simulink model "ACFT"  (R2024b)
settings: Solver=ode1  StartTime=0.0  StopTime=10.0  FixedStep=0.01  RelTol=1e-3
undefined symbols (not defined in the file): Inertia
libraries: Aerodynamics x1, Atmospheric x1, EqM x1, Propulsion x1
settings Model: Creator=ada09  LastModifiedBy=ada09
settings DataIOCC: SaveState=on  ReturnWorkspaceOutputs=off

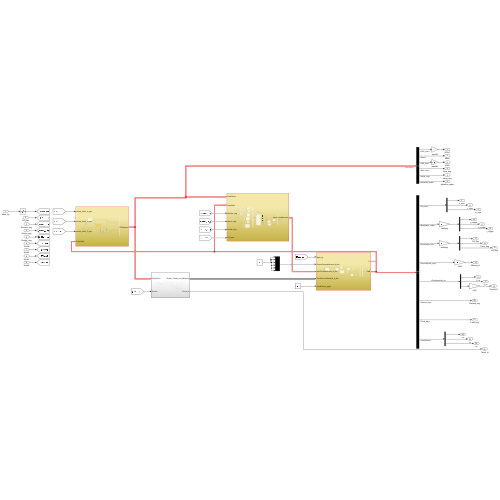
[thumbnail: Simulink's stored preview of the top-level diagram]
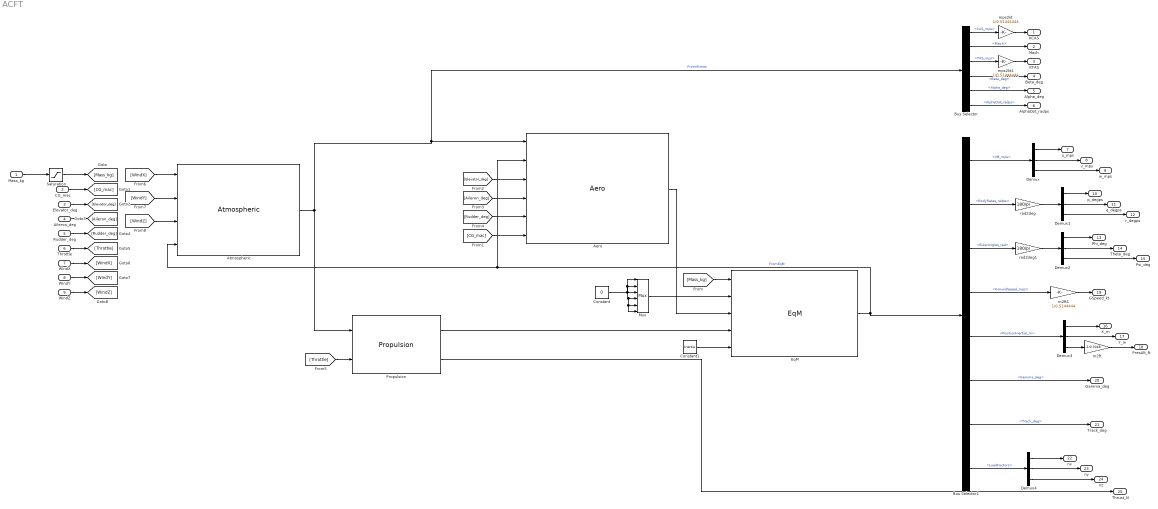
== system ACFT ==
  Mass_kg : Inport
  CG_mac : Inport  Port=2
  Elevator_deg : Inport  Port=3
  Aileron_deg : Inport  Port=4
  Rudder_deg : Inport  Port=5
  Throttle : Inport  Port=6
  WindX : Inport  Port=7
  WindY : Inport  Port=8
  WindZ : Inport  Port=9
  Aero : Aerodynamics/Aero  SystemSampleTime=-1  VariantActivationTime=update diagram  AllowFlexibleInterface=on  Latency=0  AutoFrameSizeCalculation=off
  Atmospheric : Atmospheric/Atmospheric  SystemSampleTime=-1  VariantActivationTime=update diagram  AllowFlexibleInterface=on  Latency=0  AutoFrameSizeCalculation=off
  Bus Selector : BusSelector  OutputSignals=CAS_mps,Mach,TAS_mps,Beta_deg,Alpha_deg,AlphaDot_radps
  Bus Selector1 : BusSelector  OutputSignals=VB_mps,BodyRates_radps,EulerAngles_rad,GroundSpeed_mps,PositionInertial_m,Gamma_deg,Track_deg,LoadFactors
  Constant : Constant  Value=0
  Constant1 : Constant  Value=Inertia
  Demux{,1..4} (5 alike) : Demux  Outputs=3
  EqM : EqM/EqM  SystemSampleTime=-1  VariantActivationTime=update diagram  AllowFlexibleInterface=on  Latency=0  AutoFrameSizeCalculation=off
  Mux : Mux  Inputs=6
  Propulsion : Propulsion/Propulsion  SystemSampleTime=-1  VariantActivationTime=update diagram  AllowFlexibleInterface=on  Latency=0  AutoFrameSizeCalculation=off
  Saturation : Saturate  UpperLimit=inf  LowerLimit=0.1
  m2ft : Gain  Gain=-1/0.3048
  m2ft1 : Gain  Gain=1/0.5144444
  mps2kt : Gain  Gain=1/0.51444444
  mps2kt1 : Gain  Gain=1/0.51444444
  rad2deg : Gain  Gain=180/pi
  rad2deg1 : Gain  Gain=180/pi
  KCAS : Outport
  Mach : Outport  Port=2
  KTAS : Outport  Port=3
  Beta_deg : Outport  Port=4
  "Alpha_deg " : Outport  Port=5
  AlphaDot_radps : Outport  Port=6
  u_mps : Outport  Port=7
  v_mps : Outport  Port=8
  w_mps : Outport  Port=9
  p_degps : Outport  Port=10
  q_degps : Outport  Port=11
  r_degps : Outport  Port=12
  Phi_deg : Outport  Port=13
  Theta_deg : Outport  Port=14
  Psi_deg : Outport  Port=15
  X_m : Outport  Port=16
  Y_m : Outport  Port=17
  PresAlt_ft : Outport  Port=18
  GSpeed_kt : Outport  Port=19
  Gamma_deg : Outport  Port=20
  Track_deg : Outport  Port=21
  nx : Outport  Port=22
  ny : Outport  Port=23
  nz : Outport  Port=24
  Thrust_N : Outport  Port=25
  wires:
  Atmospheric/1 -> Propulsion/1, Bus Selector/1, Aero/1  "FromAtmos"
  Propulsion/1 -> EqM/4
  EqM/1 -> Bus Selector1/1, Atmospheric/4, Aero/2  "FromEqM"
  Constant/1 -> Mux/1, Mux/6, Mux/5, Mux/4, Mux/3, Mux/2
  Mass_kg/1 -> Saturation/1
  CG_mac/1 -> [CG_mac]
  Elevator_deg/1 -> [Elevator_deg]
  Aileron_deg/1 -> [Aileron_deg]
  Rudder_deg/1 -> [Rudder_deg]
  Throttle/1 -> [Throttle]
  WindX/1 -> [WindX]
  WindY/1 -> [WindY]
  WindZ/1 -> [WindZ]
  [WindX] -> Atmospheric/1
  [WindY] -> Atmospheric/2
  [WindZ] -> Atmospheric/3
  [Throttle] -> Propulsion/2
  Constant1/1 -> EqM/5
  [CG_mac] -> Aero/6
  [Elevator_deg] -> Aero/3
  [Aileron_deg] -> Aero/4
  [Rudder_deg] -> Aero/5
  Propulsion/2 -> Thrust_N/1
  Bus Selector/1 -> mps2kt/1  "<CAS_mps>"
  Bus Selector/2 -> Mach/1  "<Mach>"
  mps2kt/1 -> KCAS/1
  Bus Selector/3 -> mps2kt1/1  "<TAS_mps>"
  mps2kt1/1 -> KTAS/1
  Bus Selector/4 -> Beta_deg/1  "<Beta_deg>"
  Bus Selector/5 -> "Alpha_deg "/1  "<Alpha_deg>"
  Bus Selector/6 -> AlphaDot_radps/1  "<AlphaDot_radps>"
  Bus Selector1/1 -> Demux/1  "<VB_mps>"
  Demux/1 -> u_mps/1
  Demux/2 -> v_mps/1
  Demux/3 -> w_mps/1
  Bus Selector1/2 -> rad2deg/1  "<BodyRates_radps>"
  rad2deg/1 -> Demux1/1
  Demux1/1 -> p_degps/1
  Demux1/2 -> q_degps/1
  Demux1/3 -> r_degps/1
  Bus Selector1/3 -> rad2deg1/1  "<EulerAngles_rad>"
  rad2deg1/1 -> Demux2/1
  Demux2/1 -> Phi_deg/1
  Demux2/2 -> Theta_deg/1
  Demux2/3 -> Psi_deg/1
  Bus Selector1/5 -> Demux3/1  "<PositionInertial_m>"
  Demux3/1 -> X_m/1
  Demux3/2 -> Y_m/1
  Demux3/3 -> m2ft/1
  m2ft/1 -> PresAlt_ft/1
  Bus Selector1/4 -> m2ft1/1  "<GroundSpeed_mps>"
  m2ft1/1 -> GSpeed_kt/1
  Bus Selector1/6 -> Gamma_deg/1  "<Gamma_deg>"
  Bus Selector1/7 -> Track_deg/1  "<Track_deg>"
  Bus Selector1/8 -> Demux4/1  "<LoadFactors>"
  Demux4/3 -> nz/1
  Demux4/1 -> nx/1
  Demux4/2 -> ny/1
  Aero/1 -> EqM/3
  Mux/1 -> EqM/2
  [Mass_kg] -> EqM/1
  Saturation/1 -> [Mass_kg]
